simulink model "ADCS_Outline"  (R2019a)
settings: Solver=VariableStepAuto  StartTime=0.0  StopTime=duration  MaxStep=step
InitFcn:
  | SC_ODIN_INITIALIZATION
values from neighbouring files (symbols this model uses):
  A = [ v(1) v(4) v(5) v(7);        v(4) v(2) v(6) v(8);        v(5) v(6) v(3) v(9);        v(7) v(8) v(9) v(10) ]    [MagnetometerCalibration.m]    (also in SC_ODIN_INITIALIZATION.m = 0.06; test.m = asin(sin(N)/sin(n)*sin(a)))
  Amag = [0.910186583854  -0.00959593267728  0.00343590491018; -0.00959593267728  1.05471221352  0.0559849466324; 0.00343590491018  0.0559849466324  1.05528532305]    [MagnetometerBias.mat]    (also in MagnetometerCalibration.m = evecs/scale*evecs')
  argentina = [1612.36;-4182.16;-4522.83]    [SC_ODIN_INITIALIZATION.m]
  As = 0.2*0.3    (= 0.06)    [SC_ODIN_INITIALIZATION.m]
  b_mag = block.InputPort(3).Data    [MagnetometerCalibration.m]    (also in SC_ODIN_INITIALIZATION.m = [10;-15.5;-12.2]*1e-6)
  bmag = [1.00003671399e-05 -1.55007781395e-05 -1.22009762149e-05]    [MagnetometerBias.mat]    (also in MagnetometerCalibration.m = centerE)
  breakpoints = data(:,1)    [SC_ODIN_INITIALIZATION.m]
  c = 2.99792458e8    (= 299792458)    [SC_ODIN_INITIALIZATION.m]
  C_I = [0.045 0.0009 -0.00007;        0.0009 0.045 -0.00003;        -0.00007 -0.00003 0.009]    [SC_ODIN_INITIALIZATION.m]
  Cd = 2.0    (= 2)    [SC_ODIN_INITIALIZATION.m]
  controller_sample_rate = 0.5    [SC_ODIN_INITIALIZATION.m]
  D = [ 2 * x,            2 * y,            2 * z,            1 + 0 * x ]    [MagnetometerCalibration.m]    (also in SC_ODIN_INITIALIZATION.m = 0.01*[1;1;1])
  datapx = data(:,2)    [SC_ODIN_INITIALIZATION.m]
  datapy = data(:,3)    [SC_ODIN_INITIALIZATION.m]
  datapz = data(:,4)    [SC_ODIN_INITIALIZATION.m]
  datavx = data(:,5)    [SC_ODIN_INITIALIZATION.m]
  datavy = data(:,6)    [SC_ODIN_INITIALIZATION.m]
  datavz = data(:,7)    [SC_ODIN_INITIALIZATION.m]
  DCM_BT0 = eye(3)    [SC_ODIN_INITIALIZATION.m]
  G = 6.67408e-11    [SC_ODIN_INITIALIZATION.m]
  ground = [1266.06;-4295.81;4526.14]    [SC_ODIN_INITIALIZATION.m]
  I = [Ixx -Ixy -Ixz;      -Ixy Iyy -Iyz;      -Ixz -Iyz Izz]    [SC_ODIN_INITIALIZATION.m]
  invA_mag = block.InputPort(2).Data    [MagnetometerCalibration.m]    (also in SC_ODIN_INITIALIZATION.m = inv(Ellrot/scale*Ellrot'))
  JD_0 = start_day+start_fraction    [SC_ODIN_INITIALIZATION.m]
  Ks = 1367    [SC_ODIN_INITIALIZATION.m]
  L = [0.0000812 -0.0022136 -0.0225868]    [SC_ODIN_INITIALIZATION.m]
  Ls = 0.01*[-3; 3; 5]    [SC_ODIN_INITIALIZATION.m]
  M = 5.9722e24    (= 5.9722e+24)    [SC_ODIN_INITIALIZATION.m]    (also in visualisation.m = uicontrol('Style','text','String',{''},'Position',[710 100+2)
  magnetorquer_tau = 0.02    [SC_ODIN_INITIALIZATION.m]
  magnetorquer_x_saturation = 0.24    [SC_ODIN_INITIALIZATION.m]
  magnetorquer_y_saturation = 0.24    [SC_ODIN_INITIALIZATION.m]
  magnetorquer_z_saturation = 0.13    [SC_ODIN_INITIALIZATION.m]
  namibia = [5659.26;1238.85;-2659.2]    [SC_ODIN_INITIALIZATION.m]
  q = 0.6    [SC_ODIN_INITIALIZATION.m]
  radii = radii .* sgns    [MagnetometerCalibration.m]    (also in SC_ODIN_INITIALIZATION.m = [1;0.9;1.1])
  W0 = [1;0;1-1/240].*pi()/180    [SC_ODIN_INITIALIZATION.m]
  wheel_saturation = 0.23e-3    (= 0.00023)    [SC_ODIN_INITIALIZATION.m]
  wheel_tau = 2    [SC_ODIN_INITIALIZATION.m]
undefined symbols (not defined in the file or in its folder): DiscIntNeverNeededParam, nut80, sun_sensors
libraries: dspmathops x94, vrlib x70, dspsrcs4 x21, realtime_pacer_lib x1, dspsolvers x1, dspinverses x1
(part 2 of 6)

== system ADCS_Outline/DISTURBANCE TORQUES/ATMOSPHERIC DRAG ==
  note: Velocity squared
  note: For h = 350 km
      |
      | Min rho = 3.17x10 E-12
      | Mean rho = 8.33x10 E-12
      | Max rho = 1.85x10 E-11
      |
      | For h = 375 km
      |
      | Min rho = 1.81x10 E-12
      | Mean rho = 5.24x10 E-12
      | Max rho = 1.25x10 E-11
      |
      | For h = 400 km
      |
      | Min rho = 1.04x10 E-12
      | Mean rho = 3.29x10 E-12
      | Max rho = 8.43x10 E-12
      |
      | Note1: Mean Rho has an accuracy of 10%
      | Note2: Rho (kg/m^3)
      | Note3 : Rho depends on solar pressure and the solar cycle
      | Source : New SMAD p.1031
  note: Atmospheric Drag
  (vx,vy,vz) : Inport
  "h " : Inport  Port=2
  Area : Constant  Value=A
  Coefficient of Drag : Constant  Value=Cd
  Constant : Constant  Value=0.5
  Cross Product : vrlib/Utilities/Cross Product
      settings: SourceProductBaseCode=VR
  Dot Product : DotProduct  InputSameDT=on  OutDataTypeStr=Inherit: Inherit via internal rule
  MATLAB Function : MATLAB Function  TreatAsAtomicUnit=on
  Multiply : Product  Inputs=6
  Product : Product  Inputs=/*
  Sqrt : Sqrt  SaturateOnIntegerOverflow=on
  "Vector from Center of Mass and Center of Aerodynamic Forces " : Constant  Value=L
  km/s to m/s : Gain  Gain=1000
  (Tax,Tay,Taz) : Outport
  wires:
  Constant/1 -> Multiply/3
  Multiply/1 -> Cross Product/1
  (vx,vy,vz)/1 -> km/s to m/s/1
  "h "/1 -> MATLAB Function/1(h)
  Sqrt/1 -> Product/1
  Product/1 -> Cross Product/2
  Dot Product/1 -> Sqrt/1, Multiply/5
  Area/1 -> Multiply/2
  Coefficient of Drag/1 -> Multiply/1
  MATLAB Function/1(rho) -> Multiply/4
  "Vector from Center of Mass and Center of Aerodynamic Forces "/1 -> Multiply/6
  Cross Product/1 -> (Tax,Tay,Taz)/1
  km/s to m/s/1 -> Dot Product/1, Product/2, Dot Product/2

== system ADCS_Outline/DISTURBANCE TORQUES/GRAVITY GRADIENT ==
  note: T = (3GM/R^5)*RbX(Ib*Rb)
      |
      | Source: SMAD and Coursera
      | University of Colorado Hanspeter
      | Schaub
  note: Gravity Gradient
  (px,py,pz) : Inport
  "(Ixx Ixy Ixz, Iyx Iyy Iyz, Izx Izy Izz)" : Inport  Port=2
  Constant2 : Constant  Value=3
  Constant5 : Constant  Value=2.5
  Cross Product1 : vrlib/Utilities/Cross Product
      settings: SourceProductBaseCode=VR
  Dot Product1 : DotProduct  InputSameDT=on  OutDataTypeStr=Inherit: Inherit via internal rule
  Gain : Gain  Gain=1000
  Gravitational Constant : Constant  Value=G*M
  Matrix Multiply : Product  Multiplication=Matrix(*)
  Power : Math  Operator=pow  SaturateOnIntegerOverflow=on
  Product1 : Product  Inputs=**/*
  (Tgx,Tgy,Tgz) : Outport
  wires:
  (px,py,pz)/1 -> Gain/1
  Dot Product1/1 -> Power/1
  Constant5/1 -> Power/2
  Cross Product1/1 -> Product1/4
  Constant2/1 -> Product1/2
  "(Ixx Ixy Ixz, Iyx Iyy Iyz, Izx Izy Izz)"/1 -> Matrix Multiply/1
  Matrix Multiply/1 -> Cross Product1/2
  Gravitational Constant/1 -> Product1/1
  Power/1 -> Product1/3
  Product1/1 -> (Tgx,Tgy,Tgz)/1
  Gain/1 -> Matrix Multiply/2, Cross Product1/1, Dot Product1/1, Dot Product1/2

== system ADCS_Outline/DISTURBANCE TORQUES/MAGNETIC FIELD  ==
  note: Magnetic Field
  (Dx,Dy,Dz) : Inport
  (Bx,By,Bz) : Inport  Port=2
  Cross Product : vrlib/Utilities/Cross Product
      settings: SourceProductBaseCode=VR
  nT to T : Gain  Gain=1e-9
  (Tmx,Tmy,Tmz) : Outport
  wires:
  Cross Product/1 -> (Tmx,Tmy,Tmz)/1
  (Bx,By,Bz)/1 -> nT to T/1
  (Dx,Dy,Dz)/1 -> Cross Product/1
  nT to T/1 -> Cross Product/2

== system ADCS_Outline/DISTURBANCE TORQUES/SOLAR RADIATION PRESSURE ==
  note: Solar Radiation
      | Pressure
  (Sx,Sy,Sz) : Inport
  Cross Product2 : vrlib/Utilities/Cross Product
      settings: SourceProductBaseCode=VR
  Inverse because the Force is in the opposite direction : Gain  Gain=-1
  Normalization : dspmathops/Normalization  NormType=2-norm  Bias=1e-10  NormOver=Each column  Dimension=1  roundingMode=Floor  overflowMode=off  accumDataTypeStr=Inherit: Same as product output  accumLastDataTypeStr=Inherit: Same as product output  outputDataTypeStr=Inherit: Same as product output  outputMin=[]  outputMax=[]  outputLastDataTypeStr=Inherit: Same as product output
      settings: SourceProductName=DSP System Toolbox
  Product3 : Product  Inputs=5
  Solar Constant : Constant  Value=Ks
  Speed of Light : Constant  Value=1/c
  Sunlit Area : Constant  Value=As
  Unitless Reflectance Factor : Constant  Value=1+q
  Vector from Center of Mass to Center of Solar Pressure : Constant  Value=Ls
  "(Tsx,Tsy, Tsz)" : Outport
  wires:
  Cross Product2/1 -> "(Tsx,Tsy, Tsz)"/1
  Sunlit Area/1 -> Product3/1
  Vector from Center of Mass to Center of Solar Pressure/1 -> Cross Product2/1
  (Sx,Sy,Sz)/1 -> Normalization/1
  Solar Constant/1 -> Product3/4
  Product3/1 -> Cross Product2/2
  Inverse because the Force is in the opposite direction/1 -> Product3/5
  Speed of Light/1 -> Product3/3
  Unitless Reflectance Factor/1 -> Product3/2
  Normalization/1 -> Inverse because the Force is in the opposite direction/1

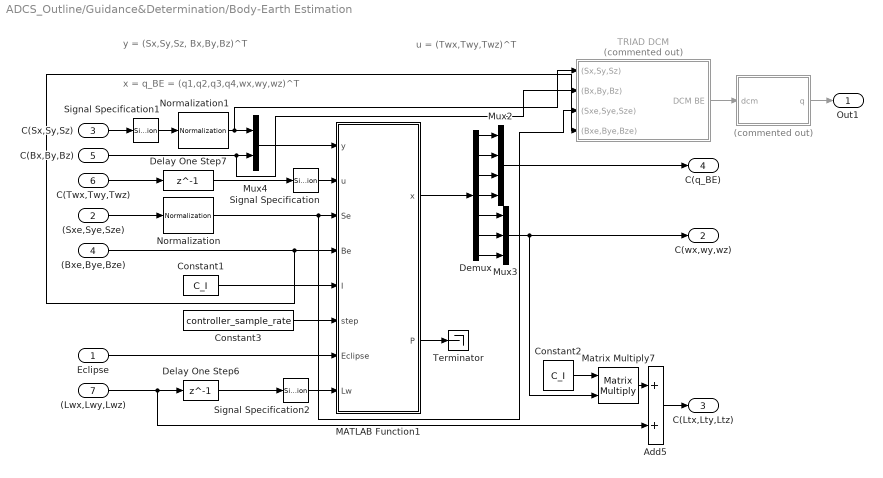
== system ADCS_Outline/Guidance&Determination/Body-Earth Estimation ==
  note: u = (Twx,Twy,Twz)^T
  note: y = (Sx,Sy,Sz, Bx,By,Bz)^T
  note: x = q_BE = (q1,q2,q3,q4,wx,wy,wz)^T
  Eclipse : Inport
  (Sxe,Sye,Sze) : Inport  Port=2
  C(Sx,Sy,Sz) : Inport  Port=3
  (Bxe,Bye,Bze) : Inport  Port=4
  C(Bx,By,Bz) : Inport  Port=5
  C(Twx,Twy,Twz) : Inport  Port=6
  (Lwx,Lwy,Lwz) : Inport  Port=7
  " " : MATLAB Function  Commented=on  TreatAsAtomicUnit=on
  Add5 : Sum
  Constant1 : Constant  Value=C_I
  Constant2 : Constant  Value=C_I
  Constant3 : Constant  Value=controller_sample_rate
  Delay One Step6 : Delay  DelayLength=1
  Delay One Step7 : Delay  DelayLength=1
  Demux : Demux  Outputs=7
  MATLAB Function1 : MATLAB Function  TreatAsAtomicUnit=on
  Matrix Multiply7 : Product  Multiplication=Matrix(*)
  Mux2 : Mux
  Mux3 : Mux  Inputs=3
  Mux4 : Mux  Inputs=2
  Normalization : dspmathops/Normalization  NormType=2-norm  Bias=1e-10  NormOver=Each column  Dimension=1  roundingMode=Floor  overflowMode=off  accumDataTypeStr=Inherit: Same as product output  accumLastDataTypeStr=Inherit: Same as product output  outputDataTypeStr=Inherit: Same as product output  outputMin=[]  outputMax=[]  outputLastDataTypeStr=Inherit: Same as product output
      settings: SourceProductName=DSP System Toolbox
  Normalization1 : dspmathops/Normalization  NormType=2-norm  Bias=1e-10  NormOver=Each column  Dimension=1  roundingMode=Floor  overflowMode=off  accumDataTypeStr=Inherit: Same as product output  accumLastDataTypeStr=Inherit: Same as product output  outputDataTypeStr=Inherit: Same as product output  outputMin=[]  outputMax=[]  outputLastDataTypeStr=Inherit: Same as product output
      settings: SourceProductName=DSP System Toolbox
  Signal Specification : SignalSpecification  Dimensions=3
  Signal Specification1 : SignalSpecification  Dimensions=3
  Signal Specification2 : SignalSpecification  Dimensions=3
  TRIAD DCM : Subsystem  Commented=on
  Terminator : Terminator
  Out1 : Outport
  C(wx,wy,wz) : Outport  Port=2
  C(Ltx,Lty,Ltz) : Outport  Port=3
  C(q_BE) : Outport  Port=4
  wires:
  Demux/4 -> Mux2/4
  Demux/3 -> Mux2/3
  Demux/2 -> Mux2/2
  Demux/1 -> Mux2/1
  Demux/5 -> Mux3/1
  Demux/6 -> Mux3/2
  Demux/7 -> Mux3/3
  Mux2/1 -> C(q_BE)/1
  Mux4/1 -> MATLAB Function1/1(y)
  C(Sx,Sy,Sz)/1 -> Signal Specification1/1
  (Sxe,Sye,Sze)/1 -> Normalization/1
  (Lwx,Lwy,Lwz)/1 -> Add5/2, Delay One Step6/1
  Add5/1 -> C(Ltx,Lty,Ltz)/1
  Constant1/1 -> MATLAB Function1/5(I)
  Matrix Multiply7/1 -> Add5/1
  Constant2/1 -> Matrix Multiply7/1
  Constant3/1 -> MATLAB Function1/6(step)
  Delay One Step6/1 -> Signal Specification2/1
  Delay One Step7/1 -> Signal Specification/1
  C(Twx,Twy,Twz)/1 -> Delay One Step7/1
  Normalization1/1 -> TRIAD DCM/1((Sx,Sy,Sz)), Mux4/1
  Normalization/1 -> TRIAD DCM/3((Sxe,Sye,Sze)), MATLAB Function1/3(Se)
  Mux3/1 -> Matrix Multiply7/2, C(wx,wy,wz)/1
  (Bxe,Bye,Bze)/1 -> TRIAD DCM/4((Bxe,Bye,Bze)), MATLAB Function1/4(Be)
  C(Bx,By,Bz)/1 -> TRIAD DCM/2(" (Bx,By,Bz)"), Mux4/2
  Eclipse/1 -> MATLAB Function1/7(Eclipse)
  MATLAB Function1/2(P) -> Terminator/1
  Signal Specification/1 -> MATLAB Function1/2(u)
  Signal Specification1/1 -> Normalization1/1
  Signal Specification2/1 -> MATLAB Function1/8(Lw)
  MATLAB Function1/1(x) -> Demux/1
  TRIAD DCM/1(DCM BE) -> " "/1(dcm)
  " "/1(q) -> Out1/1

== system ADCS_Outline/Guidance&Determination/Eclipse Prediction ==
  (Sxe,Sye,Sze) : Inport
  (Pxe,Pye,Pze) : Inport  Port=2
  Eclipse Prediction : MATLAB Function  TreatAsAtomicUnit=on
  Eclipse : Outport
  wires:
  (Sxe,Sye,Sze)/1 -> Eclipse Prediction/1(s)
  (Pxe,Pye,Pze)/1 -> Eclipse Prediction/2(p)
  Eclipse Prediction/1(Eclipse) -> Eclipse/1

== system ADCS_Outline/Guidance&Determination/Guidance ==
  Mode : Inport
  (Pxe,Pye,Pze) : Inport  Port=2
  (Vxe,Vye,Vze) : Inport  Port=3
  (Sxe,Sye,Sze) : Inport  Port=4
  C(q_BE) : Inport  Port=5
  "    " : MATLAB Function  TreatAsAtomicUnit=on
  Constant1 : Constant  Value=ground
  Constant5 : Constant  Value=argentina
  Constant6 : Constant  Value=namibia
  Guidance : MATLAB Function  TreatAsAtomicUnit=on
  TRIAD : Subsystem
  C(q_BTarget) : Outport
  qETarget : Outport  Port=2
  wires:
  (Sxe,Sye,Sze)/1 -> Guidance/2(SE)
  (Vxe,Vye,Vze)/1 -> Guidance/4(VE)
  Constant1/1 -> Guidance/7(GE)
  Constant6/1 -> Guidance/5(NE)
  Guidance/2(ConstraintE) -> TRIAD/2(ConstraintE)
  Guidance/3(PointingB) -> TRIAD/3(PointingB)
  TRIAD/1(q_ET) -> qETarget/1, "    "/2(qb)  "target"
  Constant5/1 -> Guidance/6(AE)
  Guidance/4(ConstraintB) -> TRIAD/4(ContraintB)
  Guidance/1(PointingE) -> TRIAD/1(PointingE)
  Mode/1 -> Guidance/1(Mode)  "Mode"
  (Pxe,Pye,Pze)/1 -> Guidance/3(PE)
  "    "/1(q) -> C(q_BTarget)/1
  C(q_BE)/1 -> "    "/1(qa)

== system ADCS_Outline/Guidance&Determination/Mode Selection ==
  Eclipse : Inport
  (Pxe,Pye,Pze) : Inport  Port=2
  C(Ltx,Lty,Ltz) : Inport  Port=3
  Constant : Constant  Value=ground
  Constant2 : Constant  Value=argentina
  Constant3 : Constant  Value=2
  Constant4 : Constant  Value=namibia
  Mode Selector : MATLAB Function  TreatAsAtomicUnit=on
  Mode : Outport
  wires:
  Constant/1 -> Mode Selector/3(G)
  (Pxe,Pye,Pze)/1 -> Mode Selector/5(P)
  Constant2/1 -> Mode Selector/4(A)
  Constant3/1 -> Mode Selector/1(modeOverdrive)
  Constant4/1 -> Mode Selector/2(N)
  Eclipse/1 -> Mode Selector/6(Eclipse)
  C(Ltx,Lty,Ltz)/1 -> Mode Selector/7(Ltot)
  Mode Selector/1(Mode) -> Mode/1

== system ADCS_Outline/Guidance&Determination/Rotation ==
  C(q_BE) : Inport
  (Bxe,Bye,Bze) : Inport  Port=2
  "    " : MATLAB Function  TreatAsAtomicUnit=on
  "    1" : MATLAB Function  TreatAsAtomicUnit=on
  Constant : Constant  Value=[-1 -1 -1 1]
  Demux : Demux
  MATLAB Function : MATLAB Function  TreatAsAtomicUnit=on
  Multiply : Product
  Mux : Mux  Inputs=3
  Signal Specification : SignalSpecification  Dimensions=[1 4]
  Terminator : Terminator
  C_(Bx,By,Bz) : Outport
  wires:
  Constant/1 -> Multiply/1
  C(q_BE)/1 -> Multiply/2, "    "/1(qa)
  (Bxe,Bye,Bze)/1 -> MATLAB Function/1(u)
  "    "/1(q) -> Signal Specification/1
  Multiply/1 -> "    1"/2(qb)
  MATLAB Function/1(y) -> "    "/2(qb)
  Mux/1 -> C_(Bx,By,Bz)/1
  "    1"/1(q) -> Demux/1
  Demux/1 -> Mux/1
  Demux/2 -> Mux/2
  Demux/3 -> Mux/3
  Demux/4 -> Terminator/1
  Signal Specification/1 -> "    1"/1(qa)

== system ADCS_Outline/Guidance&Determination/TargetFrameVelocity ==
  C(q_ETarget) : Inport
  "    " : MATLAB Function  TreatAsAtomicUnit=on
  Constant : Constant  Value=[1;1;1;-1]
  Demux : Demux
  Filtered Derivative1 : Subsystem
  Gain1 : Gain  Gain=2
  Multiply : Product
  Mux : Mux  Inputs=3
  Signal Specification : SignalSpecification  Dimensions=[1 4]
  Terminator : Terminator
  C(wx,wy,wz) : Outport
  wires:
  Mux/1 -> C(wx,wy,wz)/1
  Demux/4 -> Terminator/1
  Demux/3 -> Mux/3
  Demux/2 -> Mux/2
  Demux/1 -> Mux/1
  Gain1/1 -> Demux/1
  Constant/1 -> Multiply/2
  Multiply/1 -> "    "/2(qb)
  Filtered Derivative1/1(dx) -> "    "/1(qa)
  C(q_ETarget)/1 -> Multiply/1, Filtered Derivative1/1(x)
  "    "/1(q) -> Signal Specification/1
  Signal Specification/1 -> Gain1/1

== system ADCS_Outline/Magnetometer /Calibration (Calculated onboard) ==
  C(Bx,By,Bz)raw : Inport
  Mode : Inport  Port=2
  B_E : Inport  Port=3
  Add : Sum  Inputs=-+
  Bias (Hard Iron) : Constant  Value=bmag  SampleTime=-1
  Calibration : Subsystem
  Matrix Multiply : Product  Multiplication=Matrix(*)
  Stretch (Soft Iron) : Constant  Value=Amag  SampleTime=-1
  C(Bx,By,Bz)cal : Outport
  wires:
  Add/1 -> Matrix Multiply/2
  Matrix Multiply/1 -> C(Bx,By,Bz)cal/1
  Bias (Hard Iron)/1 -> Add/1
  Stretch (Soft Iron)/1 -> Matrix Multiply/1
  Mode/1 -> Calibration/2(Mode)
  C(Bx,By,Bz)raw/1 -> Calibration/1(C(Bx,By,Bz)), Add/2
  B_E/1 -> Calibration/3(B_E)

== system ADCS_Outline/Magnetometer /Noise and Bias ==
  In1 : Inport
  Add : Sum  Inputs=+++
  Bias (Hard iron) : Constant  Value=b_mag
  Matrix Multiply : Product  Multiplication=Matrix(*)
  Mux : Mux  Inputs=3
  Random Source1 : dspsrcs4/Random Source  SrcType=Gaussian  NormMethod=Ziggurat  CltLength=12  MinVal=0  MaxVal=1e-12  MeanVal=0  VarVal=(15e-9)^2  RepMode=Not repeatable  rawSeed=1  IsInherit=off  SampMode=Discrete  SampTime=controller_sample_rate  SampFrame=1  DataType=Double  OutComplex=Real  OutputFrames=off
  Random Source2 : dspsrcs4/Random Source  SrcType=Gaussian  NormMethod=Ziggurat  CltLength=12  MinVal=0  MaxVal=1e-12  MeanVal=0  VarVal=(15e-9)^2  RepMode=Not repeatable  rawSeed=1  IsInherit=off  SampMode=Discrete  SampTime=controller_sample_rate  SampFrame=1  DataType=Double  OutComplex=Real  OutputFrames=off
  Random Source3 : dspsrcs4/Random Source  SrcType=Gaussian  NormMethod=Ziggurat  CltLength=12  MinVal=0  MaxVal=1e-12  MeanVal=0  VarVal=(15e-9)^2  RepMode=Not repeatable  rawSeed=1  IsInherit=off  SampMode=Discrete  SampTime=controller_sample_rate  SampFrame=1  DataType=Double  OutComplex=Real  OutputFrames=off
  Stretch (Soft Iron) : Constant  Value=invA_mag
  loss : Gain
  Out1 : Outport
  wires:
  Bias (Hard iron)/1 -> Add/3
  Add/1 -> Out1/1
  Random Source3/1 -> Mux/3
  Random Source1/1 -> Mux/2
  Random Source2/1 -> Mux/1
  In1/1 -> loss/1
  Stretch (Soft Iron)/1 -> Matrix Multiply/1
  loss/1 -> Matrix Multiply/2
  Matrix Multiply/1 -> Add/2
  Mux/1 -> Add/1

== system ADCS_Outline/Momentum Control/Bdot Controller ==
  C(Bx,By,Bz) : Inport
  Arduino : Subsystem  Commented=on  TreatAsAtomicUnit=on
  Bang Bang Controller : Subsystem  Commented=on
  Bang Bang with direction : Subsystem  Commented=on
  Control Gain : Gain  Gain=-3e7
  Filtered Derivative : Subsystem
  Sampling rate : DiscretePulseGenerator  Commented=on  PulseType=Time based  Period=.1  PulseWidth=50
  Saturation : Subsystem
  Scope : Scope  Commented=on  NumInputPorts=2
  C(Mx,My,Mz) : Outport
  wires:
  C(Bx,By,Bz)/1 -> Filtered Derivative/1(x), Arduino/1(C(Bx,By,Bz))
  Control Gain/1 -> Saturation/1(C(Mx,My,Mz))
  Sampling rate/1 -> Arduino/Trigger
  Filtered Derivative/1(dx) -> Bang Bang with direction/1(C(Mx,My,Mz)), Bang Bang Controller/1(C(Bdotx,Bdoty,Bdotz)), Control Gain/1
  Arduino/1(C(Mx,My,Mz)) -> Scope/1
  Saturation/1(sat_C(Mx,My,Mz)) -> C(Mx,My,Mz)/1

== system ADCS_Outline/Momentum Control/Filter ==
  Noisy : Inport
  1/tau : Gain  Gain=0.05
  Add : Sum  Inputs=-+
  Discrete-Time Integrator : DiscreteIntegrator  SampleTime=-1  ICPrevOutput=DiscIntNeverNeededParam  ICPrevScaledInput=DiscIntNeverNeededParam
  Filtered : Outport
  wires:
  Add/1 -> 1/tau/1
  1/tau/1 -> Discrete-Time Integrator/1
  Noisy/1 -> Add/2
  Discrete-Time Integrator/1 -> Filtered/1, Add/1

== system ADCS_Outline/Momentum Control/Momentum Bias ==
  C(q_BE) : Inport
  (Vxe,Vye,Vze) : Inport  Port=2
  (Pxe,Pye,Pze) : Inport  Port=3
  Cross Product1 : vrlib/Utilities/Cross Product
      settings: SourceProductBaseCode=VR
  Momentum Bias : Gain  Gain=-0.5e-3
  Normalization : dspmathops/Normalization  NormType=2-norm  Bias=1e-10  NormOver=Each column  Dimension=1  roundingMode=Floor  overflowMode=off  accumDataTypeStr=Inherit: Same as product output  accumLastDataTypeStr=Inherit: Same as product output  outputDataTypeStr=Inherit: Same as product output  outputMin=[]  outputMax=[]  outputLastDataTypeStr=Inherit: Same as product output
      settings: SourceProductName=DSP System Toolbox
  Rotation : Subsystem
  C(M_B) : Outport
  wires:
  Normalization/1 -> Momentum Bias/1
  Rotation/1(vo) -> Normalization/1
  C(q_BE)/1 -> Rotation/1(q)
  Cross Product1/1 -> Rotation/2(vi)  "normal direction"
  (Pxe,Pye,Pze)/1 -> Cross Product1/2
  (Vxe,Vye,Vze)/1 -> Cross Product1/1
  Momentum Bias/1 -> C(M_B)/1

== system ADCS_Outline/Momentum Control/Saturation ==
  note: Trims the vector but keeps the same direction
  C(Mx,My,Mz) : Inport
  Demux : Demux  Outputs=3
  Divide : Product  Inputs=*/
  Max : MinMax  Function=max  Inputs=4
  Not saturated : Constant
  Saturation x : Fcn  Expr=abs(u)/magnetorquer_x_saturation
  Saturation y : Fcn  Expr=abs(u)/magnetorquer_y_saturation
  Saturation z : Fcn  Expr=abs(u)/magnetorquer_z_saturation
  sat_C(Mx,My,Mz) : Outport
  wires:
  Saturation z/1 -> Max/3
  Demux/2 -> Saturation y/1
  Max/1 -> Divide/2
  Saturation y/1 -> Max/2
  Saturation x/1 -> Max/1
  Demux/1 -> Saturation x/1
  Demux/3 -> Saturation z/1
  C(Mx,My,Mz)/1 -> Divide/1, Demux/1
  Divide/1 -> sat_C(Mx,My,Mz)/1
  Not saturated/1 -> Max/4

== system ADCS_Outline/Perfect DCM/ Imaging Argentina ==
  ToArgentina : Inport
  Constant : Constant  Value=[0;1;0]
  Constant1 : Constant  Value=[0;0;1]
  Cross Product{,1..3} (4 alike) : vrlib/Utilities/Cross Product
      settings: SourceProductBaseCode=VR
  Matrix Concatenate : Concatenate  NumInputs=3  Mode=Multidimensional array  ConcatenateDimension=2
  Matrix Concatenate1 : Concatenate  NumInputs=3  Mode=Multidimensional array  ConcatenateDimension=2
  Matrix Multiply : Product  Multiplication=Matrix(*)
  Normalization{,1..5} (6 alike) : dspmathops/Normalization  NormType=2-norm  Bias=1e-10  NormOver=Each column  Dimension=1  roundingMode=Floor  overflowMode=off  accumDataTypeStr=Inherit: Same as product output  accumLastDataTypeStr=Inherit: Same as product output  outputDataTypeStr=Inherit: Same as product output  outputMin=[]  outputMax=[]  outputLastDataTypeStr=Inherit: Same as product output
      settings: SourceProductName=DSP System Toolbox
  Signal Specification : SignalSpecification  Dimensions=3
  Signal Specification1 : SignalSpecification  Dimensions=3
  Transpose : Math  Operator=transpose  SaturateOnIntegerOverflow=on
  Velocity : Constant  Value=[1;0;0]
  DCM FN : Outport
  wires:
  Constant1/1 -> Cross Product/2
  Cross Product3/1 -> Signal Specification1/1
  Velocity/1 -> Cross Product2/2
  Normalization/1 -> Matrix Concatenate/3, Cross Product1/1
  Signal Specification1/1 -> Normalization3/1
  Signal Specification/1 -> Normalization2/1
  Matrix Multiply/1 -> DCM FN/1
  Matrix Concatenate1/1 -> Matrix Multiply/1
  Matrix Concatenate/1 -> Transpose/1
  Normalization4/1 -> Cross Product1/2, Matrix Concatenate/1
  Transpose/1 -> Matrix Multiply/2
  Cross Product2/1 -> Signal Specification/1
  Normalization1/1 -> Matrix Concatenate/2
  Cross Product/1 -> Normalization/1
  Normalization2/1 -> Matrix Concatenate1/3, Cross Product3/1
  Constant/1 -> Cross Product/1, Normalization4/1
  ToArgentina/1 -> Cross Product2/1, Normalization5/1
  Normalization3/1 -> Matrix Concatenate1/2
  Normalization5/1 -> Cross Product3/2, Matrix Concatenate1/1
  Cross Product1/1 -> Normalization1/1

== system ADCS_Outline/Perfect DCM/ Imaging Namibia ==
  ToNamibia : Inport
  Constant : Constant  Value=[0;0;1]
  Constant1 : Constant  Value=[0;1;0]
  Cross Product{,1..3} (4 alike) : vrlib/Utilities/Cross Product
      settings: SourceProductBaseCode=VR
  Matrix Concatenate : Concatenate  NumInputs=3  Mode=Multidimensional array  ConcatenateDimension=2
  Matrix Concatenate1 : Concatenate  NumInputs=3  Mode=Multidimensional array  ConcatenateDimension=2
  Matrix Multiply : Product  Multiplication=Matrix(*)
  Normalization{,1..5} (6 alike) : dspmathops/Normalization  NormType=2-norm  Bias=1e-10  NormOver=Each column  Dimension=1  roundingMode=Floor  overflowMode=off  accumDataTypeStr=Inherit: Same as product output  accumLastDataTypeStr=Inherit: Same as product output  outputDataTypeStr=Inherit: Same as product output  outputMin=[]  outputMax=[]  outputLastDataTypeStr=Inherit: Same as product output
      settings: SourceProductName=DSP System Toolbox
  Signal Specification : SignalSpecification  Dimensions=3
  Signal Specification1 : SignalSpecification  Dimensions=3
  Transpose : Math  Operator=transpose  SaturateOnIntegerOverflow=on
  Velocity : Constant  Value=[1;0;0]
  DCM FN : Outport
  wires:
  Cross Product1/1 -> Normalization1/1
  Normalization5/1 -> Matrix Concatenate1/1, Cross Product3/2
  Normalization3/1 -> Matrix Concatenate1/2
  Velocity/1 -> Normalization5/1, Cross Product2/1
  Constant/1 -> Normalization4/1, Cross Product/1
  Normalization2/1 -> Cross Product3/1, Matrix Concatenate1/3
  Cross Product/1 -> Normalization/1
  Normalization1/1 -> Matrix Concatenate/2
  Cross Product2/1 -> Signal Specification/1
  Transpose/1 -> Matrix Multiply/2
  Normalization4/1 -> Matrix Concatenate/1, Cross Product1/2
  Matrix Concatenate/1 -> Transpose/1
  Matrix Concatenate1/1 -> Matrix Multiply/1
  Matrix Multiply/1 -> DCM FN/1
  Signal Specification/1 -> Normalization2/1
  Signal Specification1/1 -> Normalization3/1
  Normalization/1 -> Cross Product1/1, Matrix Concatenate/3
  ToNamibia/1 -> Cross Product2/2
  Cross Product3/1 -> Signal Specification1/1
  Constant1/1 -> Cross Product/2

== system ADCS_Outline/Perfect DCM/ Nadir Pointing ==
  (Pv,Pw,Pr) : Inport
  Constant : Constant  Value=[0;0;1]
  Constant1 : Constant  Value=[0;-1;0]
  Cross Product{,1..3} (4 alike) : vrlib/Utilities/Cross Product
      settings: SourceProductBaseCode=VR
  Matrix Concatenate : Concatenate  NumInputs=3  Mode=Multidimensional array  ConcatenateDimension=2
  Matrix Concatenate1 : Concatenate  NumInputs=3  Mode=Multidimensional array  ConcatenateDimension=2
  Matrix Multiply : Product  Multiplication=Matrix(*)
  Normalization{,1..5} (6 alike) : dspmathops/Normalization  NormType=2-norm  Bias=1e-10  NormOver=Each column  Dimension=1  roundingMode=Floor  overflowMode=off  accumDataTypeStr=Inherit: Same as product output  accumLastDataTypeStr=Inherit: Same as product output  outputDataTypeStr=Inherit: Same as product output  outputMin=[]  outputMax=[]  outputLastDataTypeStr=Inherit: Same as product output
      settings: SourceProductName=DSP System Toolbox
  Signal Specification : SignalSpecification  Dimensions=3
  Signal Specification1 : SignalSpecification  Dimensions=3
  Transpose : Math  Operator=transpose  SaturateOnIntegerOverflow=on
  Velocity : Constant  Value=[1;0;0]
  DCM FZ : Outport
  wires:
  Constant1/1 -> Cross Product/2
  Cross Product3/1 -> Signal Specification1/1
  (Pv,Pw,Pr)/1 -> Cross Product2/2
  Normalization/1 -> Matrix Concatenate/3, Cross Product1/1
  Signal Specification1/1 -> Normalization3/1
  Signal Specification/1 -> Normalization2/1
  Matrix Multiply/1 -> DCM FZ/1
  Matrix Concatenate1/1 -> Matrix Multiply/1
  Matrix Concatenate/1 -> Transpose/1
  Normalization4/1 -> Cross Product1/2, Matrix Concatenate/1
  Transpose/1 -> Matrix Multiply/2
  Cross Product2/1 -> Signal Specification/1
  Normalization1/1 -> Matrix Concatenate/2
  Cross Product/1 -> Normalization/1
  Normalization2/1 -> Matrix Concatenate1/3, Cross Product3/1
  Constant/1 -> Cross Product/1, Normalization4/1
  Velocity/1 -> Cross Product2/1, Normalization5/1
  Normalization3/1 -> Matrix Concatenate1/2
  Normalization5/1 -> Cross Product3/2, Matrix Concatenate1/1
  Cross Product1/1 -> Normalization1/1

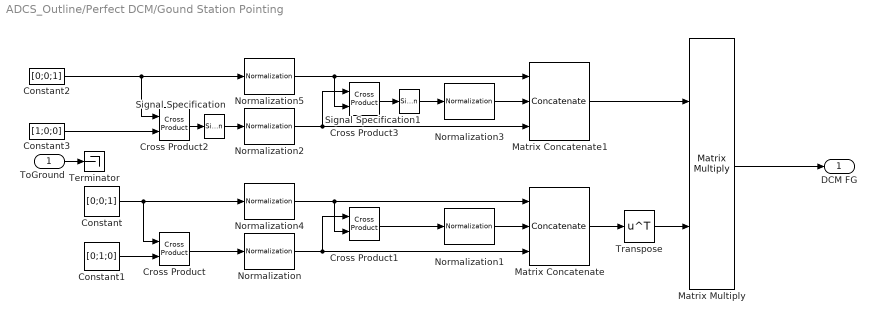
== system ADCS_Outline/Perfect DCM/Gound Station Pointing ==
  ToGround : Inport
  Constant : Constant  Value=[0;0;1]
  Constant1 : Constant  Value=[0;1;0]
  Constant2 : Constant  Value=[0;0;1]
  Constant3 : Constant  Value=[1;0;0]
  Cross Product{,1..3} (4 alike) : vrlib/Utilities/Cross Product
      settings: SourceProductBaseCode=VR
  Matrix Concatenate : Concatenate  NumInputs=3  Mode=Multidimensional array  ConcatenateDimension=2
  Matrix Concatenate1 : Concatenate  NumInputs=3  Mode=Multidimensional array  ConcatenateDimension=2
  Matrix Multiply : Product  Multiplication=Matrix(*)
  Normalization{,1..5} (6 alike) : dspmathops/Normalization  NormType=2-norm  Bias=1e-10  NormOver=Each column  Dimension=1  roundingMode=Floor  overflowMode=off  accumDataTypeStr=Inherit: Same as product output  accumLastDataTypeStr=Inherit: Same as product output  outputDataTypeStr=Inherit: Same as product output  outputMin=[]  outputMax=[]  outputLastDataTypeStr=Inherit: Same as product output
      settings: SourceProductName=DSP System Toolbox
  Signal Specification : SignalSpecification  Dimensions=3
  Signal Specification1 : SignalSpecification  Dimensions=3
  Terminator : Terminator
  Transpose : Math  Operator=transpose  SaturateOnIntegerOverflow=on
  DCM FG : Outport
  wires:
  Cross Product1/1 -> Normalization1/1
  Normalization5/1 -> Matrix Concatenate1/1, Cross Product3/2
  Normalization3/1 -> Matrix Concatenate1/2
  Constant2/1 -> Normalization5/1, Cross Product2/1
  Constant/1 -> Normalization4/1, Cross Product/1
  Normalization2/1 -> Cross Product3/1, Matrix Concatenate1/3
  Cross Product/1 -> Normalization/1
  Normalization1/1 -> Matrix Concatenate/2
  Cross Product2/1 -> Signal Specification/1
  Transpose/1 -> Matrix Multiply/2
  Normalization4/1 -> Matrix Concatenate/1, Cross Product1/2
  Matrix Concatenate/1 -> Transpose/1
  Matrix Concatenate1/1 -> Matrix Multiply/1
  Matrix Multiply/1 -> DCM FG/1
  Signal Specification/1 -> Normalization2/1
  Signal Specification1/1 -> Normalization3/1
  Normalization/1 -> Cross Product1/1, Matrix Concatenate/3
  Constant3/1 -> Cross Product2/2
  Cross Product3/1 -> Signal Specification1/1
  Constant1/1 -> Cross Product/2
  ToGround/1 -> Terminator/1

== system ADCS_Outline/Perfect DCM/Sun Pointing ==
  (Sv,Sw,Sr) : Inport
  Constant : Constant  Value=[1;-1;0]
  Constant1 : Constant  Value=[0;0;1]
  Constant2 : Constant  Value=[1;0;0]
  Constant3 : Constant  Value=[-1;-1;0]
  Cross Product{,1..3} (4 alike) : vrlib/Utilities/Cross Product
      settings: SourceProductBaseCode=VR
  Fcn : Fcn  Expr=u(2)
  Matrix Concatenate : Concatenate  NumInputs=3  Mode=Multidimensional array  ConcatenateDimension=2
  Matrix Concatenate1 : Concatenate  NumInputs=3  Mode=Multidimensional array  ConcatenateDimension=2
  Matrix Multiply : Product  Multiplication=Matrix(*)
  Normalization{,1..5} (6 alike) : dspmathops/Normalization  NormType=2-norm  Bias=1e-10  NormOver=Each column  Dimension=1  roundingMode=Floor  overflowMode=off  accumDataTypeStr=Inherit: Same as product output  accumLastDataTypeStr=Inherit: Same as product output  outputDataTypeStr=Inherit: Same as product output  outputMin=[]  outputMax=[]  outputLastDataTypeStr=Inherit: Same as product output
      settings: SourceProductName=DSP System Toolbox
  Signal Specification1 : SignalSpecification  Dimensions=3
  Switch : Switch  Criteria=u2 > Threshold
  Transpose : Math  Operator=transpose  SaturateOnIntegerOverflow=on
  DCM FS : Outport
  wires:
  Normalization/1 -> Cross Product1/1, Matrix Concatenate/3
  Normalization5/1 -> Matrix Concatenate1/1, Cross Product3/2
  Cross Product1/1 -> Normalization1/1
  Normalization3/1 -> Matrix Concatenate1/2
  Cross Product3/1 -> Signal Specification1/1
  Constant1/1 -> Cross Product/2
  Normalization4/1 -> Matrix Concatenate/1, Cross Product1/2
  Switch/1 -> Normalization4/1, Cross Product/1
  Cross Product2/1 -> Normalization2/1
  Cross Product/1 -> Normalization/1
  Normalization1/1 -> Matrix Concatenate/2
  Normalization2/1 -> Cross Product3/1, Matrix Concatenate1/3
  Matrix Concatenate/1 -> Transpose/1
  Matrix Concatenate1/1 -> Matrix Multiply/1
  Transpose/1 -> Matrix Multiply/2
  (Sv,Sw,Sr)/1 -> Fcn/1, Cross Product2/1, Normalization5/1
  Constant2/1 -> Cross Product2/2
  Signal Specification1/1 -> Normalization3/1
  Matrix Multiply/1 -> DCM FS/1
  Constant/1 -> Switch/3
  Constant3/1 -> Switch/1
  Fcn/1 -> Switch/2

== system ADCS_Outline/Reaction Wheels/Torque Saturation ==
  note: Trims the vector but keeps the same direction
  C(Twx,Twy,Twz) : Inport
  Demux : Demux  Outputs=3
  Divide : Product  Inputs=*/
  Max : MinMax  Function=max  Inputs=4  ZeroCross=off
  Not saturated : Constant
  Saturation x : Fcn  Expr=abs(u)/wheel_saturation
  Saturation y : Fcn  Expr=abs(u)/wheel_saturation
  Saturation z : Fcn  Expr=abs(u)/wheel_saturation
  sat_C(Twx,Twy,Twz) : Outport
  wires:
  Saturation z/1 -> Max/3
  Demux/2 -> Saturation y/1
  Divide/1 -> sat_C(Twx,Twy,Twz)/1
  Max/1 -> Divide/2
  Saturation y/1 -> Max/2
  C(Twx,Twy,Twz)/1 -> Divide/1, Demux/1
  Saturation x/1 -> Max/1
  Demux/1 -> Saturation x/1
  Demux/3 -> Saturation z/1
  Not saturated/1 -> Max/4

== system ADCS_Outline/Reaction Wheels Control/Filtered Derivative ==
  x : Inport
  Add : Sum  Inputs=-+
  Discrete-Time Integrator : DiscreteIntegrator  SampleTime=-1  ICPrevOutput=DiscIntNeverNeededParam  ICPrevScaledInput=DiscIntNeverNeededParam
  Time Constant (1/tau) : Gain
  dx : Outport
  wires:
  Discrete-Time Integrator/1 -> Add/1
  Time Constant (1/tau)/1 -> Discrete-Time Integrator/1, dx/1
  Add/1 -> Time Constant (1/tau)/1
  x/1 -> Add/2

== system ADCS_Outline/Reaction Wheels Control/Torque Saturation ==
  note: Trims the vector but keeps the same direction
  C(Twx,Twy,Twz) : Inport
  Demux : Demux  Outputs=3
  Divide : Product  Inputs=*/
  Max : MinMax  Function=max  Inputs=4  ZeroCross=off
  Not saturated : Constant
  Saturation x : Fcn  Expr=abs(u)/(0.9*wheel_saturation)
  Saturation y : Fcn  Expr=abs(u)/(0.9*wheel_saturation)
  Saturation z : Fcn  Expr=abs(u)/(0.9*wheel_saturation)
  sat_C(Twx,Twy,Twz) : Outport
  wires:
  Saturation z/1 -> Max/3
  Demux/2 -> Saturation y/1
  Divide/1 -> sat_C(Twx,Twy,Twz)/1
  Max/1 -> Divide/2
  Saturation y/1 -> Max/2
  C(Twx,Twy,Twz)/1 -> Divide/1, Demux/1
  Saturation x/1 -> Max/1
  Demux/1 -> Saturation x/1
  Demux/3 -> Saturation z/1
  Not saturated/1 -> Max/4

== system ADCS_Outline/S//C Kinematics/Skewed ==
  v : Inport
  MATLAB Function : MATLAB Function  TreatAsAtomicUnit=on
  m : Outport
  wires:
  v/1 -> MATLAB Function/1(u)
  MATLAB Function/1(y) -> m/1

== system ADCS_Outline/STK Attitude Recording/Subsystem ==
  q_EB : Inport
  Trigger : TriggerPort  VariantControl=Variant  PortDimensions=1
  To Workspace : ToWorkspace  VariableName=q_EB  SampleTime=-1
  wires:
  q_EB/1 -> To Workspace/1

== system ADCS_Outline/Sun Sensors/Noise and Bias ==
  In1 : Inport
  Add : Sum  Inputs=+++
  Bias : Constant  Commented=on  Value=0.1*[1;1;1;1;1;1;1;1;1;1;1;1]
  Mux : Mux  Inputs=3
  Random Source : dspsrcs4/Random Source  SrcType=Gaussian  NormMethod=Ziggurat  CltLength=12  MinVal=0  MaxVal=1  MeanVal=0  VarVal=1e-5  RepMode=Not repeatable  rawSeed=1  IsInherit=off  SampMode=Discrete  SampTime=controller_sample_rate  SampFrame=1  DataType=Double  OutComplex=Real  OutputFrames=off
  Random Source1 : dspsrcs4/Random Source  SrcType=Gaussian  NormMethod=Ziggurat  CltLength=12  MinVal=0  MaxVal=1  MeanVal=0  VarVal=1e-5  RepMode=Not repeatable  rawSeed=1  IsInherit=off  SampMode=Discrete  SampTime=controller_sample_rate  SampFrame=1  DataType=Double  OutComplex=Real  OutputFrames=off
  Random Source2 : dspsrcs4/Random Source  SrcType=Gaussian  NormMethod=Ziggurat  CltLength=12  MinVal=0  MaxVal=1  MeanVal=0  VarVal=1e-5  RepMode=Not repeatable  rawSeed=1  IsInherit=off  SampMode=Discrete  SampTime=controller_sample_rate  SampFrame=1  DataType=Double  OutComplex=Real  OutputFrames=off
  loss : Gain
  Out1 : Outport
  wires:
  Random Source1/1 -> Mux/2
  Random Source2/1 -> Mux/3
  Random Source/1 -> Mux/1
  Bias/1 -> Add/3
  Mux/1 -> Add/1
  Add/1 -> loss/1
  In1/1 -> Add/2
  loss/1 -> Out1/1

== system ADCS_Outline/Toolbox/DCM2W ==
  note: [C]dot=-w[C]
  DCM : Inport
  Anti-Skewed : Subsystem
  Filtered Derivative : Subsystem
  Gain1 : Gain  Gain=-1
  Matrix Multiply1 : Product  Multiplication=Matrix(*)
  Signal Specification : SignalSpecification  Dimensions=3
  Transpose1 : Math  Operator=transpose  SaturateOnIntegerOverflow=on
  W : Outport
  wires:
  Transpose1/1 -> Matrix Multiply1/2
  Matrix Multiply1/1 -> Gain1/1
  Gain1/1 -> Anti-Skewed/1(m)
  DCM/1 -> Transpose1/1, Filtered Derivative/1(x)
  Anti-Skewed/1(v) -> Signal Specification/1
  Filtered Derivative/1(dx) -> Matrix Multiply1/1
  Signal Specification/1 -> W/1

== system ADCS_Outline/Toolbox/Decoder ==
  note: for the analog sun sensors
  C(sensors readings) : Inport
  Constant : Constant  Value=sun_sensors
  LU Solver : dspsolvers/LU Solver
      settings: SourceProductName=DSP System Toolbox  SourceProductBaseCode=DS
  MATLAB Function1 : MATLAB Function  TreatAsAtomicUnit=on
  C(Sx,Sy,Sz) : Outport
  wires:
  MATLAB Function1/2(B) -> LU Solver/2
  C(sensors readings)/1 -> MATLAB Function1/1(readings)
  MATLAB Function1/1(A) -> LU Solver/1
  Constant/1 -> MATLAB Function1/2(vectors)
  LU Solver/1 -> C(Sx,Sy,Sz)/1

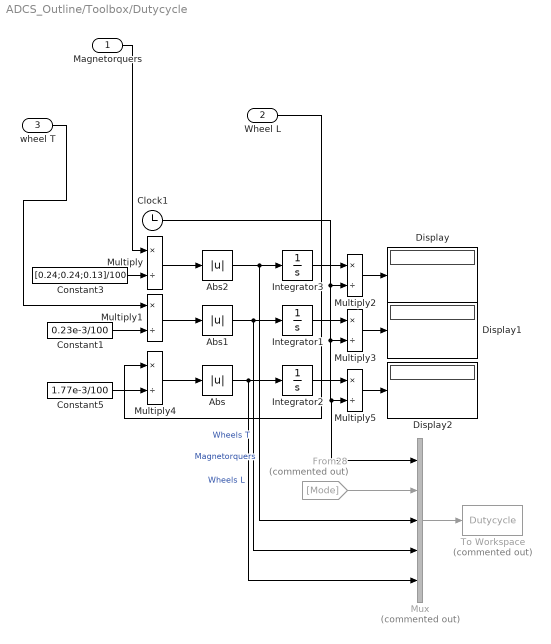
== system ADCS_Outline/Toolbox/Dutycycle ==
  Magnetorquers : Inport
  Wheel L : Inport  Port=2
  wheel T : Inport  Port=3
  Abs : Abs
  Abs1 : Abs
  Abs2 : Abs
  Clock1 : Clock
  Constant1 : Constant  Value=0.23e-3/100
  Constant3 : Constant  Value=[0.24;0.24;0.13]/100
  Constant5 : Constant  Value=1.77e-3/100
  Display : Display
  Display1 : Display
  Display2 : Display
  From28 : From  Commented=on  GotoTag=Mode
  Integrator1 : Integrator
  Integrator2 : Integrator
  Integrator3 : Integrator
  Multiply{,1..5} (6 alike) : Product  Inputs=*/
  Mux : Mux  Commented=on  Inputs=5
  To Workspace : ToWorkspace  Commented=on  VariableName=Dutycycle  SampleTime=-1
  wires:
  Integrator2/1 -> Multiply5/1
  Constant3/1 -> Multiply/2
  Multiply/1 -> Abs2/1
  Constant5/1 -> Multiply4/2
  Abs1/1 -> Mux/4, Integrator1/1  "Wheels T"
  Wheel L/1 -> Multiply4/1
  Multiply1/1 -> Abs1/1
  Abs2/1 -> Mux/3, Integrator3/1  "Magnetorquers"
  Clock1/1 -> Mux/1, Multiply5/2, Multiply3/2, Multiply2/2
  Integrator3/1 -> Multiply2/1
  Constant1/1 -> Multiply1/2
  Multiply2/1 -> Display/1
  Multiply3/1 -> Display1/1
  Multiply4/1 -> Abs/1
  From28/1 -> Mux/2
  Integrator1/1 -> Multiply3/1
  Abs/1 -> Mux/5, Integrator2/1  "Wheels L"
  Mux/1 -> To Workspace/1
  Multiply5/1 -> Display2/1
  wheel T/1 -> Multiply1/1
  Magnetorquers/1 -> Multiply/1

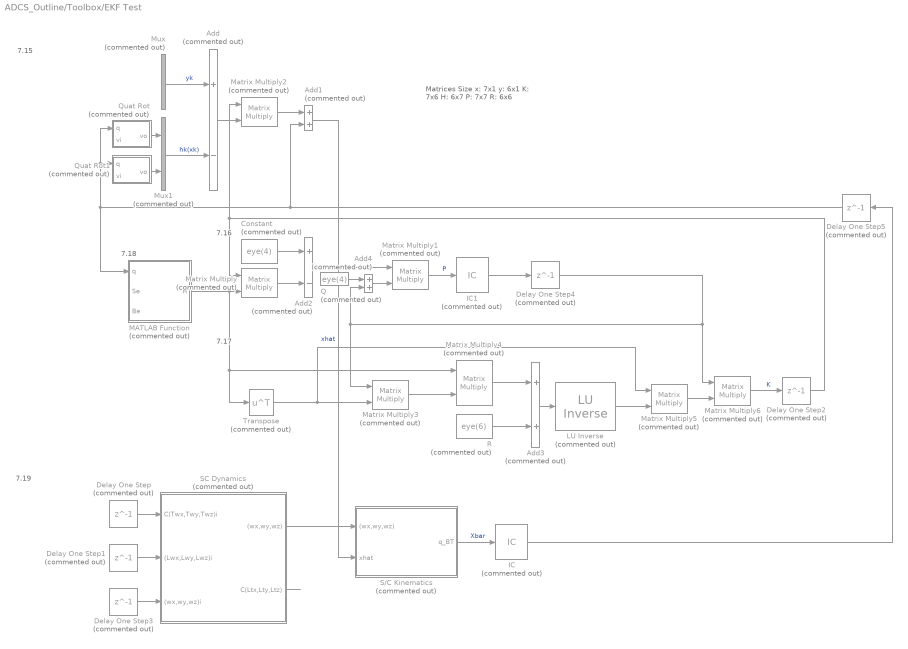
== system ADCS_Outline/Toolbox/EKF Test ==
  note: 7.19
  note: Matrices Size
      |
      | x: 7x1
      | y: 6x1
      | K: 7x6
      | H: 6x7
      | P: 7x7
      | R: 6x6
  note: 7.17
  note: 7.16
  note: 7.18
  note: 7.15
  " LU Inverse" : dspinverses/ LU Inverse  Commented=on
      settings: SourceProductName=DSP System Toolbox
  Add : Sum  Commented=on  Inputs=+-
  Add1 : Sum  Commented=on
  Add2 : Sum  Commented=on  Inputs=+-
  Add3 : Sum  Commented=on
  Add4 : Sum  Commented=on
  Constant : Constant  Commented=on  Value=eye(4)
  Delay One Step{,1..5} (6 alike) : Delay  Commented=on  DelayLength=1
  IC : InitialCondition  Commented=on  Value=[0;0;0;1]
  IC1 : InitialCondition  Commented=on  Value=eye(4)
  MATLAB Function : MATLAB Function  Commented=on  TreatAsAtomicUnit=on
  Matrix Multiply{,1..6} (7 alike) : Product  Commented=on  Multiplication=Matrix(*)
  Mux : Mux  Commented=on  Inputs=2
  Mux1 : Mux  Commented=on  Inputs=2
  Q : Constant  Commented=on  Value=eye(4)
  Quat Rot : Subsystem  Commented=on
  Quat Rot1 : Subsystem  Commented=on
  R : Constant  Commented=on  Value=eye(6)
  S/C Kinematics : Subsystem  Commented=on
  SC Dynamics : Subsystem  Commented=on
  Transpose : Math  Commented=on  Operator=transpose  SaturateOnIntegerOverflow=on
  wires:
  ? -> Delay One Step/1
  Add4/1 -> Matrix Multiply1/2
  Delay One Step2/1 -> Matrix Multiply2/1, Matrix Multiply/1
  Mux1/1 -> Add/2  "hk(xk)"
  Delay One Step4/1 -> Matrix Multiply6/1, Add4/2, Matrix Multiply3/1
  S/C Kinematics/1(q_BT) -> IC/1  "Xbar"
  Add1/1 -> S/C Kinematics/2(xhat)  "xhat"
  IC/1 -> Delay One Step5/1
  Matrix Multiply4/1 -> Add3/1
  Delay One Step/1 -> SC Dynamics/1(C(Twx,Twy,Twz)i)
  ? -> Delay One Step1/1
  SC Dynamics/1((wx,wy,wz)) -> S/C Kinematics/1((wx,wy,wz))
  Mux/1 -> Add/1  "yk"
  Add/1 -> Matrix Multiply2/2
  Matrix Multiply6/1 -> Delay One Step2/1  "K"
  Delay One Step5/1 -> Add1/2, Quat Rot1/1(q), Quat Rot/1(q), MATLAB Function/1(q)
  Delay One Step1/1 -> SC Dynamics/2((Lwx,Lwy,Lwz)i)
  MATLAB Function/1(H) -> Transpose/1, Matrix Multiply4/1, Matrix Multiply/2
  Transpose/1 -> Matrix Multiply5/1, Matrix Multiply3/2
  ? -> MATLAB Function/2(Se)
  Q/1 -> Add4/1
  Matrix Multiply3/1 -> Matrix Multiply4/2
  Quat Rot1/1(vo) -> Mux1/2
  " LU Inverse"/1 -> Matrix Multiply5/2
  Quat Rot/1(vo) -> Mux1/1
  Constant/1 -> Add2/1
  Delay One Step3/1 -> SC Dynamics/3((wx,wy,wz)i)
  Matrix Multiply/1 -> Add2/2
  Add2/1 -> Matrix Multiply1/1
  R/1 -> Add3/2
  Matrix Multiply1/1 -> IC1/1  "P"
  SC Dynamics/2(C(Ltx,Lty,Ltz)) -> ?
  ? -> Mux/1
  Matrix Multiply2/1 -> Add1/1
  ? -> Quat Rot1/2(vi)
  Matrix Multiply5/1 -> Matrix Multiply6/2
  Add3/1 -> " LU Inverse"/1
  ? -> MATLAB Function/3(Be)
  ? -> Mux/2
  ? -> Quat Rot/2(vi)
  IC1/1 -> Delay One Step4/1

== system ADCS_Outline/Toolbox/Filter ==
  Noisy : Inport
  1/tau : Gain  Gain=0.1
  Add : Sum  Inputs=-+
  Discrete-Time Integrator : DiscreteIntegrator  SampleTime=-1  ICPrevOutput=DiscIntNeverNeededParam  ICPrevScaledInput=DiscIntNeverNeededParam
  Filtered : Outport
  wires:
  Add/1 -> 1/tau/1
  1/tau/1 -> Discrete-Time Integrator/1
  Noisy/1 -> Add/2
  Discrete-Time Integrator/1 -> Filtered/1, Add/1

== system ADCS_Outline/Toolbox/No Control fast STK attitude recoding ==
  V_E : Inport
  S_E : Inport  Port=2
  P_E : Inport  Port=3
  "   DCM EF" : Subsystem
  Constant : Constant  Value=ground
  Constant2 : Constant  Value=argentina
  Constant4 : Constant  Value=namibia
  Mode Selector : MATLAB Function  TreatAsAtomicUnit=on
  Perfect DCM1 : Subsystem
  STK Attitude Recording1 : Subsystem  StopFcn=STKAttitudeFileGenerator
  wires:
  Mode Selector/1(Mode) -> Perfect DCM1/4(mode), STK Attitude Recording1/2(Mode)
  Constant2/1 -> Mode Selector/2(A)
  P_E/1 -> "   DCM EF"/2((Pxe,Pye,Pze)), Perfect DCM1/3((Pxe,Pye,Pze)), Mode Selector/1(P)
  S_E/1 -> Perfect DCM1/2((Sxe,Sye,Sze))
  Perfect DCM1/1(DCM TargetE) -> STK Attitude Recording1/1(DCM_BE)
  Constant4/1 -> Mode Selector/3(N)
  Constant/1 -> Mode Selector/4(G)
  V_E/1 -> "   DCM EF"/1((Vxe,Xye,Vze))
  "   DCM EF"/1(DCM EF) -> Perfect DCM1/1("DCM_EF ")

== system ADCS_Outline/Toolbox/Noise and Bias ==
  In1 : Inport
  Add : Sum  Inputs=+++
  Bias : Constant  Commented=on  Value=0.1*[1;1;1;1;1;1;1;1;1;1;1;1]
  Mux : Mux  Commented=on  Inputs=12
  Random Source{,1..11} (12 alike) : dspsrcs4/Random Source  Commented=on  SrcType=Gaussian  NormMethod=Ziggurat  CltLength=12  MinVal=0  MaxVal=1  MeanVal=0  VarVal=1e-4  RepMode=Not repeatable  rawSeed=1  IsInherit=off  SampMode=Discrete  SampTime=controller_sample_rate  SampFrame=1  DataType=Double  OutComplex=Real  OutputFrames=off
  loss : Gain
  Out1 : Outport
  wires:
  loss/1 -> Out1/1
  In1/1 -> Add/2
  Add/1 -> loss/1
  Mux/1 -> Add/1
  Bias/1 -> Add/3
  Random Source/1 -> Mux/1
  Random Source11/1 -> Mux/12
  Random Source10/1 -> Mux/11
  Random Source9/1 -> Mux/10
  Random Source8/1 -> Mux/9
  Random Source7/1 -> Mux/8
  Random Source6/1 -> Mux/7
  Random Source5/1 -> Mux/6
  Random Source4/1 -> Mux/5
  Random Source3/1 -> Mux/4
  Random Source2/1 -> Mux/3
  Random Source1/1 -> Mux/2

== system ADCS_Outline/Toolbox/Prediction covariance tester1 ==
  Tw : Inport
  w : Inport  Port=2
  lw : Inport  Port=3
  q : Inport  Port=4
  Add1 : Sum  Inputs=-+
  Constant : Constant  Value=controller_sample_rate
  Constant1 : Constant  Value=(C_I)
  Delay One Step2 : Delay  DelayLength=1
  Display : Display
  MATLAB Function : MATLAB Function  TreatAsAtomicUnit=on
  Mux : Mux  Inputs=2
  Mux1 : Mux  Inputs=2
  Scope : Scope  NumInputPorts=2
  To Workspace : ToWorkspace  VariableName=error  SampleTime=-1
  wires:
  Mux/1 -> Add1/1
  Add1/1 -> To Workspace/1, Display/1
  MATLAB Function/2(predictionw) -> Mux1/2
  MATLAB Function/1(predictionq) -> Mux1/1
  Mux1/1 -> Delay One Step2/1
  q/1 -> MATLAB Function/1(qi), Scope/1, Mux/1
  w/1 -> MATLAB Function/2(wi), Mux/2
  Tw/1 -> MATLAB Function/6(u)
  Constant/1 -> MATLAB Function/3(step)
  lw/1 -> MATLAB Function/5(Lw)  "Wheel L"
  Constant1/1 -> MATLAB Function/4(I)
  Delay One Step2/1 -> Scope/2, Add1/2

== system ADCS_Outline/Toolbox/Quat Rot ==
  q : Inport
  vi : Inport  Port=2
  "    " : MATLAB Function  TreatAsAtomicUnit=on
  "    1" : MATLAB Function  TreatAsAtomicUnit=on
  Constant : Constant  Value=[-1 -1 -1 1]
  Demux : Demux
  MATLAB Function : MATLAB Function  TreatAsAtomicUnit=on
  Multiply : Product
  Mux : Mux  Inputs=3
  Terminator : Terminator
  vo : Outport
  wires:
  Constant/1 -> Multiply/1
  q/1 -> Multiply/2, "    "/1(qa)
  vi/1 -> MATLAB Function/1(u)
  "    "/1(q) -> "    1"/1(qa)
  Multiply/1 -> "    1"/2(qb)
  MATLAB Function/1(y) -> "    "/2(qb)
  Mux/1 -> vo/1
  "    1"/1(q) -> Demux/1
  Demux/1 -> Mux/1
  Demux/2 -> Mux/2
  Demux/3 -> Mux/3
  Demux/4 -> Terminator/1

== system ADCS_Outline/Toolbox/S//C Kinematics1 ==
  (wx,wy,wz) : Inport
  " " : MATLAB Function  TreatAsAtomicUnit=on
  Constant : Constant  Value=[-1;-1;-1;1]
  Constant1 : Constant  Value=[-1;-1;-1;1]
  Gain1 : Gain  Gain=0.5
  Initial attitude : Constant  Value=DCM_BT0
  Integrator : Integrator  InitialConditionSource=external
  MATLAB Function1 : MATLAB Function  Commented=on  TreatAsAtomicUnit=on
  Matrix Multiply : Product  Multiplication=Matrix(*)
  Multiply : Product
  Multiply1 : Product
  Skewed : Subsystem
  q_BT : Outport
  wires:
  Skewed/1(m) -> Matrix Multiply/1
  Initial attitude/1 -> " "/1(dcm)
  Integrator/1 -> Gain1/1, Multiply/2
  Gain1/1 -> Matrix Multiply/2
  (wx,wy,wz)/1 -> Skewed/1(v)
  Matrix Multiply/1 -> Integrator/1
  Multiply/1 -> q_BT/1
  Constant/1 -> Multiply/1
  Constant1/1 -> Multiply1/1
  " "/1(q) -> Multiply1/2
  Multiply1/1 -> Integrator/2

== system ADCS_Outline/Toolbox/S//C Kinematics2 ==
  (wx,wy,wz) : Inport
  " " : MATLAB Function  TreatAsAtomicUnit=on
  Constant : Constant  Value=[-1;-1;-1;1]
  Constant1 : Constant  Value=[-1;-1;-1;1]
  Gain1 : Gain  Gain=0.5
  Initial attitude : Constant  Value=DCM_BT0
  Integrator : Integrator  InitialConditionSource=external
  MATLAB Function1 : MATLAB Function  Commented=on  TreatAsAtomicUnit=on
  Matrix Multiply : Product  Multiplication=Matrix(*)
  Multiply : Product
  Multiply1 : Product
  Skewed : Subsystem
  q_BT : Outport
  wires:
  Skewed/1(m) -> Matrix Multiply/1
  Initial attitude/1 -> " "/1(dcm)
  Integrator/1 -> Gain1/1, Multiply/2
  Gain1/1 -> Matrix Multiply/2
  (wx,wy,wz)/1 -> Skewed/1(v)
  Matrix Multiply/1 -> Integrator/1
  Multiply/1 -> q_BT/1
  Constant/1 -> Multiply/1
  Constant1/1 -> Multiply1/1
  " "/1(q) -> Multiply1/2
  Multiply1/1 -> Integrator/2

== system ADCS_Outline/Toolbox/TRIAD DCM ==
  (Sx,Sy,Sz) : Inport
  " (Bx,By,Bz)" : Inport  Port=2
  (Sxe,Sye,Sze) : Inport  Port=3
  (Bxe,Bye,Bze) : Inport  Port=4
  Cross Product{,1..3} (4 alike) : vrlib/Utilities/Cross Product
      settings: SourceProductBaseCode=VR
  Matrix Concatenate : Concatenate  NumInputs=3  Mode=Multidimensional array  ConcatenateDimension=2
  Matrix Concatenate1 : Concatenate  NumInputs=3  Mode=Multidimensional array  ConcatenateDimension=2
  Matrix Multiply : Product  Multiplication=Matrix(*)
  Normalization{,1..5} (6 alike) : dspmathops/Normalization  NormType=2-norm  Bias=1e-10  NormOver=Each column  Dimension=1  roundingMode=Floor  overflowMode=off  accumDataTypeStr=Inherit: Same as product output  accumLastDataTypeStr=Inherit: Same as product output  outputDataTypeStr=Inherit: Same as product output  outputMin=[]  outputMax=[]  outputLastDataTypeStr=Inherit: Same as product output
      settings: SourceProductName=DSP System Toolbox
  Signal Specification1 : SignalSpecification  Dimensions=3
  Transpose : Math  Operator=transpose  SaturateOnIntegerOverflow=on
  DCM BE : Outport
  wires:
  Normalization/1 -> Matrix Concatenate/3, Cross Product1/1
  Normalization5/1 -> Matrix Concatenate1/1, Cross Product3/2
  Cross Product1/1 -> Normalization1/1
  Normalization3/1 -> Matrix Concatenate1/2
  Cross Product3/1 -> Signal Specification1/1
  (Bxe,Bye,Bze)/1 -> Cross Product/2
  Normalization4/1 -> Matrix Concatenate/1, Cross Product1/2
  (Sxe,Sye,Sze)/1 -> Normalization4/1, Cross Product/1
  Cross Product2/1 -> Normalization2/1
  Cross Product/1 -> Normalization/1
  Normalization1/1 -> Matrix Concatenate/2
  Normalization2/1 -> Cross Product3/1, Matrix Concatenate1/3
  Matrix Concatenate/1 -> Transpose/1
  Matrix Concatenate1/1 -> Matrix Multiply/1
  Transpose/1 -> Matrix Multiply/2
  (Sx,Sy,Sz)/1 -> Cross Product2/1, Normalization5/1
  " (Bx,By,Bz)"/1 -> Cross Product2/2
  Matrix Multiply/1 -> DCM BE/1
  Signal Specification1/1 -> Normalization3/1

== system ADCS_Outline/wheel speed feedback/Noise and Bias ==
  In1 : Inport
  Add : Sum  Inputs=+++
  Bias : Constant  Commented=on  Value=0.1*[1;1;1;1;1;1;1;1;1;1;1;1]
  Mux : Mux  Inputs=3
  Random Source1 : dspsrcs4/Random Source  SrcType=Gaussian  NormMethod=Ziggurat  CltLength=12  MinVal=0  MaxVal=1e-12  MeanVal=0  VarVal=1.36e-13  RepMode=Not repeatable  rawSeed=1  IsInherit=off  SampMode=Discrete  SampTime=controller_sample_rate  SampFrame=1  DataType=Double  OutComplex=Real  OutputFrames=off
  Random Source2 : dspsrcs4/Random Source  SrcType=Gaussian  NormMethod=Ziggurat  CltLength=12  MinVal=0  MaxVal=1e-12  MeanVal=0  VarVal=1.36e-13  RepMode=Not repeatable  rawSeed=1  IsInherit=off  SampMode=Discrete  SampTime=controller_sample_rate  SampFrame=1  DataType=Double  OutComplex=Real  OutputFrames=off
  Random Source3 : dspsrcs4/Random Source  SrcType=Gaussian  NormMethod=Ziggurat  CltLength=12  MinVal=0  MaxVal=1e-12  MeanVal=0  VarVal=1.36e-13  RepMode=Not repeatable  rawSeed=1  IsInherit=off  SampMode=Discrete  SampTime=controller_sample_rate  SampFrame=1  DataType=Double  OutComplex=Real  OutputFrames=off
  loss : Gain
  Out1 : Outport
  wires:
  In1/1 -> Add/2
  Add/1 -> loss/1
  Bias/1 -> Add/3
  loss/1 -> Out1/1
  Random Source3/1 -> Mux/3
  Random Source1/1 -> Mux/2
  Random Source2/1 -> Mux/1
  Mux/1 -> Add/1
